simulink model "assortedStateflowElements"  (R2025a)
settings: Solver=VariableStepAuto  StartTime=0.0  StopTime=10.0  RelTol=1e-3
settings Model: Creator=willager  LastModifiedBy=willager

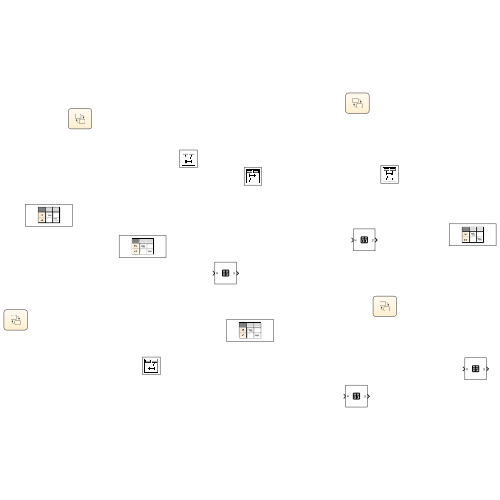
[thumbnail: Simulink's stored preview of the top-level diagram]
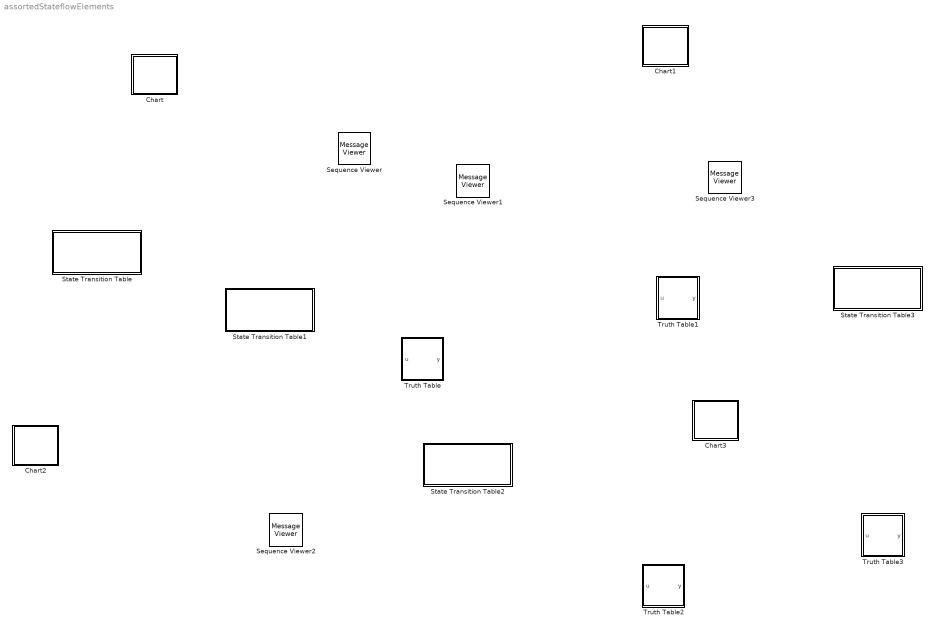
== system assortedStateflowElements ==
  Chart : Stateflow chart  TreatAsAtomicUnit=on
  Chart1 : Stateflow chart  TreatAsAtomicUnit=on
  Chart2 : Stateflow chart  TreatAsAtomicUnit=on
  Chart3 : Stateflow chart  TreatAsAtomicUnit=on
  Sequence Viewer{,1..3} (4 alike) : MessageViewer
  State Transition Table : State Transition Table  TreatAsAtomicUnit=on
  State Transition Table1 : State Transition Table  TreatAsAtomicUnit=on
  State Transition Table2 : State Transition Table  TreatAsAtomicUnit=on
  State Transition Table3 : State Transition Table  TreatAsAtomicUnit=on
  Truth Table : Truth Table  TreatAsAtomicUnit=on
  Truth Table1 : Truth Table  TreatAsAtomicUnit=on
  Truth Table2 : Truth Table  TreatAsAtomicUnit=on
  Truth Table3 : Truth Table  TreatAsAtomicUnit=on

== matlab function assortedStateflowElements/Truth Table3 ==
  data: u input; y output
function y = fcn(u)

aVarTruthTableCondition_1 = false;
aVarTruthTableCondition_2 = false;


% Example condition 1

aVarTruthTableCondition_1 = logical(u >= 0);

% Example condition 2

aVarTruthTableCondition_2 = logical(u ^ 2 <= 1);

if (aVarTruthTableCondition_1 && aVarTruthTableCondition_2)
    aFcnTruthTableAction_1();
elseif (~aVarTruthTableCondition_1 && ~aVarTruthTableCondition_2)
    aFcnTruthTableAction_1();
else % Default
    aFcnTruthTableAction_2();
end

function aFcnTruthTableAction_1()

% Example action 1 called from D1 & D2 column in condition table

y = u;

function aFcnTruthTableAction_2()

% Example action 2 called from D3 column in condition table

y = 1 / u;

== stateflow chart assortedStateflowElements/Chart1 ==

== matlab function assortedStateflowElements/Truth Table ==
  data: u input; y output
function y = fcn(u)

aVarTruthTableCondition_1 = false;
aVarTruthTableCondition_2 = false;


% Example condition 1

aVarTruthTableCondition_1 = logical(u >= 0);

% Example condition 2

aVarTruthTableCondition_2 = logical(u ^ 2 <= 1);

if (aVarTruthTableCondition_1 && aVarTruthTableCondition_2)
    aFcnTruthTableAction_1();
elseif (~aVarTruthTableCondition_1 && ~aVarTruthTableCondition_2)
    aFcnTruthTableAction_1();
else % Default
    aFcnTruthTableAction_2();
end

function aFcnTruthTableAction_1()

% Example action 1 called from D1 & D2 column in condition table

y = u;

function aFcnTruthTableAction_2()

% Example action 2 called from D3 column in condition table

y = 1 / u;

== stateflow chart assortedStateflowElements/Chart ==

== stateflow chart assortedStateflowElements/State Transition Table ==
  state state1
  state state2
  (default) -> state1
  state1 -> state2

== matlab function assortedStateflowElements/Truth Table1 ==
  data: u input; y output
function y = fcn(u)

aVarTruthTableCondition_1 = false;
aVarTruthTableCondition_2 = false;


% Example condition 1

aVarTruthTableCondition_1 = logical(u >= 0);

% Example condition 2

aVarTruthTableCondition_2 = logical(u ^ 2 <= 1);

if (aVarTruthTableCondition_1 && aVarTruthTableCondition_2)
    aFcnTruthTableAction_1();
elseif (~aVarTruthTableCondition_1 && ~aVarTruthTableCondition_2)
    aFcnTruthTableAction_1();
else % Default
    aFcnTruthTableAction_2();
end

function aFcnTruthTableAction_1()

% Example action 1 called from D1 & D2 column in condition table

y = u;

function aFcnTruthTableAction_2()

% Example action 2 called from D3 column in condition table

y = 1 / u;

== stateflow chart assortedStateflowElements/State Transition Table1 ==
  state state1
  state state2
  (default) -> state1
  state1 -> state2

== stateflow chart assortedStateflowElements/Chart2 ==

== stateflow chart assortedStateflowElements/State Transition Table2 ==
  state state1
  state state2
  (default) -> state1
  state1 -> state2

== matlab function assortedStateflowElements/Truth Table2 ==
  data: u input; y output
function y = fcn(u)

aVarTruthTableCondition_1 = false;
aVarTruthTableCondition_2 = false;


% Example condition 1

aVarTruthTableCondition_1 = logical(u >= 0);

% Example condition 2

aVarTruthTableCondition_2 = logical(u ^ 2 <= 1);

if (aVarTruthTableCondition_1 && aVarTruthTableCondition_2)
    aFcnTruthTableAction_1();
elseif (~aVarTruthTableCondition_1 && ~aVarTruthTableCondition_2)
    aFcnTruthTableAction_1();
else % Default
    aFcnTruthTableAction_2();
end

function aFcnTruthTableAction_1()

% Example action 1 called from D1 & D2 column in condition table

y = u;

function aFcnTruthTableAction_2()

% Example action 2 called from D3 column in condition table

y = 1 / u;

== stateflow chart assortedStateflowElements/Chart3 ==

== stateflow chart assortedStateflowElements/State Transition Table3 ==
  state state1
  state state2
  (default) -> state1
  state1 -> state2
